simulink model "gm_spectrum_analyser"  (R2020a)
settings: Solver=VariableStepAuto  StartTime=0.0  StopTime=100000/256e6  RelTol=1e-3
InitFcn:
  | fs = 256e6;
undefined symbols (not defined in the file or in its folder): designMultirateFIR
libraries: hdlsllib x81, simulink x50, dspmlti4 x6, dsphdlxfrm x5, hdlmdlgenlib x4, dspswit3 x4, dspsigops x2, dspsigattribs x2
(part 1 of 5)
settings Model: Creator=david  LastModifiedBy=kevin
settings OptimizationCC: BlockReduction=off  ConditionallyExecuteInputs=off  DefaultParameterBehavior=Inlined
settings DebuggingCC: AlgebraicLoopMsg=error  InheritedTsInSrcMsg=none
settings HardwareCC: ProdBitPerPointer=32  ProdBitPerSizeT=32  ProdBitPerPtrDiffT=32  ProdLargestAtomicFloat=None  ProdIntDivRoundTo=Undefined  ProdEndianess=Unspecified  ProdWordSize=32  ProdHWDeviceType=ASIC/FPGA->ASIC/FPGA  TargetBitPerPointer=64  TargetBitPerSizeT=64  TargetBitPerPtrDiffT=64  TargetLongLongMode=on  TargetIntDivRoundTo=Zero  TargetEndianess=LittleEndian  TargetWordSize=64  TargetHWDeviceType=Custom Processor->MATLAB Host Computer  ProdEqTarget=off

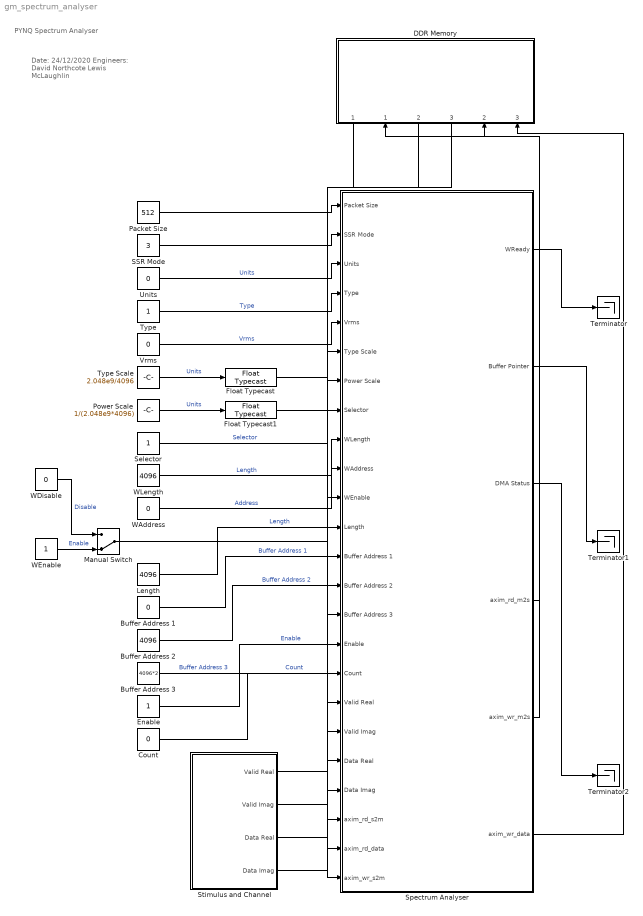
== system gm_spectrum_analyser ==
  note: PYNQ Spectrum Analyser
  note: Date:		24/12/2020
      | Engineers:	David Northcote
      | 			Lewis McLaughlin
  Buffer Address 1 : Constant  Value=0  OutDataTypeStr=uint32  SampleTime=1/fs
  Buffer Address 2 : Constant  Value=4096  OutDataTypeStr=uint32  SampleTime=1/fs
  Buffer Address 3 : Constant  Value=4096*2  OutDataTypeStr=uint32  SampleTime=1/fs
  Count : Constant  Value=0  OutDataTypeStr=uint32  SampleTime=1/fs
  DDR Memory : Subsystem
      settings: PortSchema="{\"entries\":[{\"content\":{\"sides\":[{\"content\":{\"connectorIds\":[]},\"type\":\"ConnectorPlacement.EquallySpacedRectSide\",\"uuid\":\"d9e4a1d3-1a90-455f-8481-c9ba23695512\"},{\"content\":{\"connectorIds\":[],\"side\":\"RIGHT\"},\"type\":\"ConnectorPlacement.EquallySpacedRectSide\",\"uuid\":\"d5cbf6c4-ca28-4b6e-a385-26c8d45a1027\"},{\"content\":{\"connectorIds\":[],\"side\":\"TOP\"},\"type\":\"ConnectorPlacement.EquallySpacedRectSide\",\"uuid\":\"1f61d25a-c781-4c7b-9600-adf853a1e7e2\"},{\"content\":{\"connectorIds\":[\"Out1\",\"In1\",\"Out2\",\"Out3\",\"In2\",\"In3\"],\"side\":\"BOTTOM\"},\"type\":\"ConnectorPlacement.EquallySpacedRectSide\",\"uuid\":\"b1131089-25c6-4639-a5ae-8f8dd9cc5fb0\"}]},\"type\":\"ConnectorPlacement.EquallySpacedConnector\",\"uuid\":\"baa6cdf8-4ad4-4b76-ad8b-23012dfe0a1e\"}],\"packageUris\":[\"http://schema.mathworks.com/mf0/Connector/19700101\"],\"version\":\"1.0\"}"
  Enable : Constant  OutDataTypeStr=uint32  SampleTime=1/fs
  Float Typecast : FloatTypecast
  Float Typecast1 : FloatTypecast
  Length : Constant  Value=4096  OutDataTypeStr=uint32  SampleTime=1/fs
  Manual Switch : ManualSwitch  CurrentSetting=0
  Packet Size : Constant  Value=512  OutDataTypeStr=uint32  SampleTime=-1
  Power Scale : Constant  Value=1/(2.048e9*4096)  OutDataTypeStr=single  SampleTime=-1
  SSR Mode : Constant  Value=3  OutDataTypeStr=uint32  SampleTime=-1
  Selector : Constant  OutDataTypeStr=uint32  SampleTime=-1
  Spectrum Analyser : Subsystem  TreatAsAtomicUnit=on
  Stimulus and Channel : Subsystem
  Terminator : Terminator
  Terminator1 : Terminator
  Terminator2 : Terminator
  Type : Constant  OutDataTypeStr=uint32  SampleTime=-1
  Type Scale : Constant  Value=2.048e9/4096  OutDataTypeStr=single  SampleTime=-1
  Units : Constant  Value=0  OutDataTypeStr=uint32  SampleTime=-1
  Vrms : Constant  Value=0  OutDataTypeStr=uint32  SampleTime=-1
  WAddress : Constant  Value=0  OutDataTypeStr=uint32  SampleTime=1/fs
  WDisable : Constant  Value=0  OutDataTypeStr=uint32  SampleTime=1/fs
  WEnable : Constant  OutDataTypeStr=uint32  SampleTime=1/fs
  WLength : Constant  Value=4096  OutDataTypeStr=uint32  SampleTime=1/fs
  wires:
  Spectrum Analyser/3(DMA Status) -> Terminator2/1
  Spectrum Analyser/2(Buffer Pointer) -> Terminator1/1
  Spectrum Analyser/1(WReady) -> Terminator/1
  Count/1 -> Spectrum Analyser/17(Count)  "Count"
  Enable/1 -> Spectrum Analyser/16(Enable)  "Enable"
  Buffer Address 2/1 -> Spectrum Analyser/14(Buffer Address 2)  "Buffer Address 2"
  Buffer Address 3/1 -> Spectrum Analyser/15(Buffer Address 3)  "Buffer Address 3"
  Buffer Address 1/1 -> Spectrum Analyser/13(Buffer Address 1)  "Buffer Address 1"
  Length/1 -> Spectrum Analyser/12(Length)  "Length"
  DDR Memory/3(axim_wr_s2m) -> Spectrum Analyser/24(axim_wr_s2m)
  DDR Memory/2(axim_rd_data) -> Spectrum Analyser/23(axim_rd_data)
  DDR Memory/1(axim_rd_s2m) -> Spectrum Analyser/22(axim_rd_s2m)
  Spectrum Analyser/6(axim_wr_data) -> DDR Memory/3(axim_wr_data)
  Spectrum Analyser/5(axim_wr_m2s) -> DDR Memory/2(axim_wr_m2s)
  Spectrum Analyser/4(axim_rd_m2s) -> DDR Memory/1(axim_rd_m2s)
  WLength/1 -> Spectrum Analyser/9(WLength)  "Length"
  WAddress/1 -> Spectrum Analyser/10(WAddress)  "Address"
  Manual Switch/1 -> Spectrum Analyser/11(WEnable)
  WDisable/1 -> Manual Switch/1  "Disable"
  WEnable/1 -> Manual Switch/2  "Enable"
  Packet Size/1 -> Spectrum Analyser/1(Packet Size)
  SSR Mode/1 -> Spectrum Analyser/2(SSR Mode)
  Selector/1 -> Spectrum Analyser/8(Selector)  "Selector"
  Power Scale/1 -> Float Typecast1/1  "Units"
  Float Typecast1/1 -> Spectrum Analyser/7(Power Scale)
  Float Typecast/1 -> Spectrum Analyser/6(Type Scale)
  Type Scale/1 -> Float Typecast/1  "Units"
  Units/1 -> Spectrum Analyser/3(Units)  "Units"
  Type/1 -> Spectrum Analyser/4(Type)  "Type"
  Vrms/1 -> Spectrum Analyser/5(Vrms)  "Vrms"
  Stimulus and Channel/4(Data Imag) -> Spectrum Analyser/21(Data Imag)
  Stimulus and Channel/3(Data Real) -> Spectrum Analyser/20(Data Real)
  Stimulus and Channel/2(Valid Imag) -> Spectrum Analyser/19(Valid Imag)
  Stimulus and Channel/1(Valid Real) -> Spectrum Analyser/18(Valid Real)

== system gm_spectrum_analyser/DDR Memory ==
  axim_rd_m2s : Inport
  axim_wr_m2s : Inport  Port=2
  axim_wr_data : Inport  Port=3
  AXI Read Interface Response Model : Subsystem
      settings: PortSchema="{\"entries\":[{\"content\":{\"sides\":[{\"content\":{\"connectorIds\":[]},\"type\":\"ConnectorPlacement.EquallySpacedRectSide\",\"uuid\":\"2b557e1e-8026-43d3-80e6-d6d80e534d60\"},{\"content\":{\"connectorIds\":[\"Out1\",\"In1\",\"Out2\"],\"side\":\"RIGHT\"},\"type\":\"ConnectorPlacement.EquallySpacedRectSide\",\"uuid\":\"d37ff7b5-bcab-46eb-bf2f-7b890d421095\"},{\"content\":{\"connectorIds\":[],\"side\":\"TOP\"},\"type\":\"ConnectorPlacement.EquallySpacedRectSide\",\"uuid\":\"b7392330-958c-44c2-9b9d-e2e6efc00005\"}]},\"type\":\"ConnectorPlacement.EquallySpacedConnector\",\"uuid\":\"d6fedbd7-9a1a-42de-85f8-78943e8230da\"}],\"packageUris\":[\"http://schema.mathworks.com/mf0/Connector/19700101\"],\"version\":\"1.0\"}"
  AXI Write Interface Response Model : Subsystem
      settings: PortSchema="{\"entries\":[{\"content\":{\"sides\":[{\"content\":{\"connectorIds\":[]},\"type\":\"ConnectorPlacement.EquallySpacedRectSide\",\"uuid\":\"6953abbe-a6d5-4686-b276-b89fe5e6bb23\"},{\"content\":{\"connectorIds\":[],\"side\":\"RIGHT\"},\"type\":\"ConnectorPlacement.EquallySpacedRectSide\",\"uuid\":\"539ff6ac-c243-4534-87d0-888ff9534a8b\"},{\"content\":{\"connectorIds\":[],\"side\":\"TOP\"},\"type\":\"ConnectorPlacement.EquallySpacedRectSide\",\"uuid\":\"8a126ba7-8eec-4733-ae4d-1ac2504ae558\"},{\"content\":{\"connectorIds\":[\"Out1\",\"In1\",\"In2\"],\"side\":\"BOTTOM\"},\"type\":\"ConnectorPlacement.EquallySpacedRectSide\",\"uuid\":\"05254abb-7168-4864-8cc1-53a55061df5a\"}]},\"type\":\"ConnectorPlacement.EquallySpacedConnector\",\"uuid\":\"821e8dd7-bdc5-437f-b697-1dcc78127ace\"}],\"packageUris\":[\"http://schema.mathworks.com/mf0/Connector/19700101\"],\"version\":\"1.0\"}"
  axim_rd_s2m : Outport
  axim_rd_data : Outport  Port=2
  axim_wr_s2m : Outport  Port=3
  wires:
  axim_wr_data/1 -> AXI Write Interface Response Model/2(axim_wr_data)
  AXI Read Interface Response Model/2(axim_rd_s2m) -> axim_rd_s2m/1  "axim_rd_s2m"
  axim_rd_m2s/1 -> AXI Read Interface Response Model/1(axim_rd_m2s)
  AXI Write Interface Response Model/1(axim_wr_s2m) -> axim_wr_s2m/1
  AXI Read Interface Response Model/1(axim_rd_data) -> axim_rd_data/1  "axim_rd_data"
  axim_wr_m2s/1 -> AXI Write Interface Response Model/1(axim_wr_m2s)

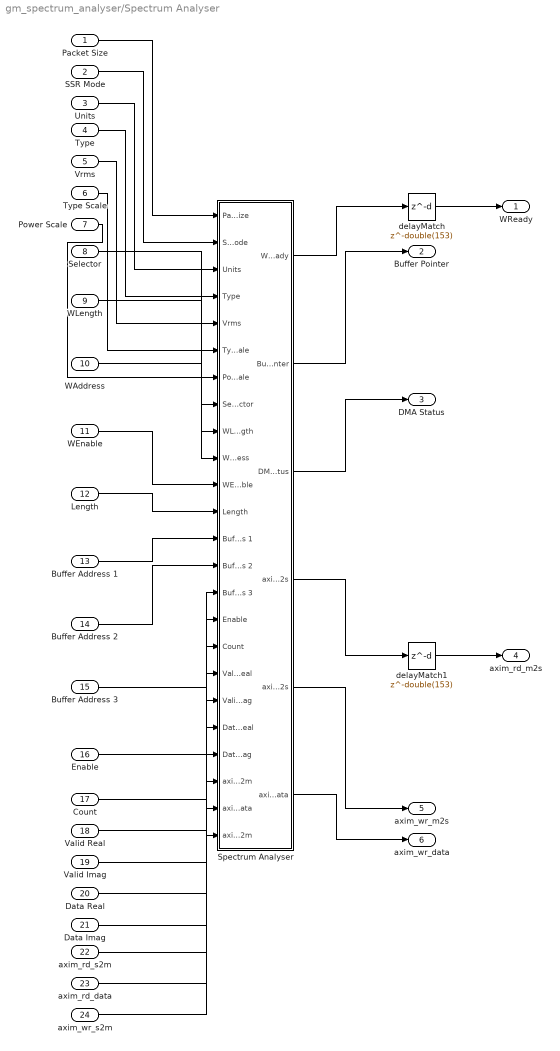
== system gm_spectrum_analyser/Spectrum Analyser ==
  Packet Size : Inport  OutDataTypeStr=uint32  PortDimensions=1  SampleTime=3.90625e-09
  SSR Mode : Inport  Port=2  OutDataTypeStr=uint32  PortDimensions=1  SampleTime=3.90625e-09
  Units : Inport  Port=3  OutDataTypeStr=uint32  PortDimensions=1  SampleTime=3.90625e-09
  Type : Inport  Port=4  OutDataTypeStr=uint32  PortDimensions=1  SampleTime=3.90625e-09
  Vrms : Inport  Port=5  OutDataTypeStr=uint32  PortDimensions=1  SampleTime=3.90625e-09
  Type Scale : Inport  Port=6  OutDataTypeStr=uint32  PortDimensions=1  SampleTime=3.90625e-09
  Power Scale : Inport  Port=7  OutDataTypeStr=uint32  PortDimensions=1  SampleTime=3.90625e-09
  Selector : Inport  Port=8  OutDataTypeStr=uint32  PortDimensions=1  SampleTime=3.90625e-09
  WLength : Inport  Port=9  OutDataTypeStr=uint32  PortDimensions=1  SampleTime=3.90625e-09
  WAddress : Inport  Port=10  OutDataTypeStr=uint32  PortDimensions=1  SampleTime=3.90625e-09
  WEnable : Inport  Port=11  OutDataTypeStr=uint32  PortDimensions=1  SampleTime=3.90625e-09
  Length : Inport  Port=12  OutDataTypeStr=uint32  PortDimensions=1  SampleTime=3.90625e-09
  Buffer Address 1 : Inport  Port=13  OutDataTypeStr=uint32  PortDimensions=1  SampleTime=3.90625e-09
  Buffer Address 2 : Inport  Port=14  OutDataTypeStr=uint32  PortDimensions=1  SampleTime=3.90625e-09
  Buffer Address 3 : Inport  Port=15  OutDataTypeStr=uint32  PortDimensions=1  SampleTime=3.90625e-09
  Enable : Inport  Port=16  OutDataTypeStr=uint32  PortDimensions=1  SampleTime=3.90625e-09
  Count : Inport  Port=17  OutDataTypeStr=uint32  PortDimensions=1  SampleTime=3.90625e-09
  Valid Real : Inport  Port=18  OutDataTypeStr=boolean  PortDimensions=1  SampleTime=3.90625e-09
  Valid Imag : Inport  Port=19  OutDataTypeStr=boolean  PortDimensions=1  SampleTime=3.90625e-09
  Data Real : Inport  Port=20  OutDataTypeStr=fixdt(0, 128, 0)  PortDimensions=1  SampleTime=3.90625e-09
  Data Imag : Inport  Port=21  OutDataTypeStr=fixdt(0, 128, 0)  PortDimensions=1  SampleTime=3.90625e-09
  axim_rd_s2m : Inport  Port=22  SampleTime=3.90625e-09
  axim_rd_data : Inport  Port=23  OutDataTypeStr=uint16  PortDimensions=1  SampleTime=3.90625e-09
  axim_wr_s2m : Inport  Port=24  SampleTime=3.90625e-09
  Spectrum Analyser : Subsystem
  delayMatch : Delay  DelayLength=double(153)  InitialCondition=0  SampleTime=3.90625e-09
  delayMatch1 : Delay  DelayLength=double(153)  InitialCondition=0  SampleTime=3.90625e-09
  WReady : Outport
  Buffer Pointer : Outport  Port=2
  DMA Status : Outport  Port=3
  axim_rd_m2s : Outport  Port=4
  axim_wr_m2s : Outport  Port=5
  axim_wr_data : Outport  Port=6
  wires:
  Packet Size/1 -> Spectrum Analyser/1(Packet Size)
  SSR Mode/1 -> Spectrum Analyser/2(SSR Mode)
  Units/1 -> Spectrum Analyser/3(Units)
  Type/1 -> Spectrum Analyser/4(Type)
  Vrms/1 -> Spectrum Analyser/5(Vrms)
  Type Scale/1 -> Spectrum Analyser/6(Type Scale)
  Power Scale/1 -> Spectrum Analyser/7(Power Scale)
  Selector/1 -> Spectrum Analyser/8(Selector)
  WLength/1 -> Spectrum Analyser/9(WLength)
  WAddress/1 -> Spectrum Analyser/10(WAddress)
  WEnable/1 -> Spectrum Analyser/11(WEnable)
  Length/1 -> Spectrum Analyser/12(Length)
  Buffer Address 1/1 -> Spectrum Analyser/13(Buffer Address 1)
  Buffer Address 2/1 -> Spectrum Analyser/14(Buffer Address 2)
  Buffer Address 3/1 -> Spectrum Analyser/15(Buffer Address 3)
  Enable/1 -> Spectrum Analyser/16(Enable)
  Count/1 -> Spectrum Analyser/17(Count)
  Valid Real/1 -> Spectrum Analyser/18(Valid Real)
  Valid Imag/1 -> Spectrum Analyser/19(Valid Imag)
  Data Real/1 -> Spectrum Analyser/20(Data Real)
  Data Imag/1 -> Spectrum Analyser/21(Data Imag)
  axim_rd_s2m/1 -> Spectrum Analyser/22(axim_rd_s2m)
  axim_rd_data/1 -> Spectrum Analyser/23(axim_rd_data)
  axim_wr_s2m/1 -> Spectrum Analyser/24(axim_wr_s2m)
  delayMatch/1 -> WReady/1
  Spectrum Analyser/2(Buffer Pointer) -> Buffer Pointer/1
  Spectrum Analyser/3(DMA Status) -> DMA Status/1
  delayMatch1/1 -> axim_rd_m2s/1
  Spectrum Analyser/5(axim_wr_m2s) -> axim_wr_m2s/1
  Spectrum Analyser/6(axim_wr_data) -> axim_wr_data/1
  Spectrum Analyser/1(WReady) -> delayMatch/1
  Spectrum Analyser/4(axim_rd_m2s) -> delayMatch1/1

== system gm_spectrum_analyser/Stimulus and Channel ==
  Channel : Subsystem
  Enable : Constant  OutDataTypeStr=boolean  SampleTime=-1
  Transmitter : Subsystem  TreatAsAtomicUnit=on
  Value : Constant  Value=hex2dec('7FFF7FFF')  OutDataTypeStr=uint32  SampleTime=-1
  Valid Real : Outport
  Valid Imag : Outport  Port=2
  Data Real : Outport  Port=3
  Data Imag : Outport  Port=4
  wires:
  Channel/2(Data Real) -> Data Real/1
  Channel/1(Valid Real) -> Valid Real/1
  Channel/4(Data Imag) -> Data Imag/1
  Channel/3(Valid Imag) -> Valid Imag/1
  Value/1 -> Transmitter/2(Value)  "Value"
  Transmitter/2(Data) -> Channel/2(Data)
  Transmitter/1(Valid) -> Channel/1(Valid)
  Enable/1 -> Transmitter/1(Enable)  "Enable"

== system gm_spectrum_analyser/DDR Memory/AXI Read Interface Response Model ==
  axim_rd_m2s : Inport
  Bus Creator : BusCreator  Inputs=2
  Bus Selector : BusSelector  OutputSignals=rd_addr,rd_len,rd_avalid
  Constant3 : Constant  OutDataTypeStr=boolean  SampleTime=-1
  DDR : Subsystem  mask{DDR_DATA=uint16(ones(1,4096)*2^15)}
      mask init:
      | %load('ram_data');
  axim_rd_data : Outport  VectorParamsAs1DForOutWhenUnconnected=off
  axim_rd_s2m : Outport  Port=2  VectorParamsAs1DForOutWhenUnconnected=off
  wires:
  Bus Creator/1 -> axim_rd_s2m/1
  DDR/1(rd_data) -> axim_rd_data/1  "rd_data"
  DDR/3(rd_dvalid) -> Bus Creator/2  "rd_dvalid"
  Constant3/1 -> DDR/4(rd_ready)
  Bus Selector/1 -> DDR/1(rd_addr)  "<rd_addr>"
  axim_rd_m2s/1 -> Bus Selector/1
  Bus Selector/3 -> DDR/3(rd_avalid)  "<rd_avalid>"
  DDR/2(rd_aready) -> Bus Creator/1  "rd_aready"
  Bus Selector/2 -> DDR/2(rd_len)  "<rd_len>"

== system gm_spectrum_analyser/DDR Memory/AXI Write Interface Response Model ==
  axim_wr_m2s : Inport
  axim_wr_data : Inport  Port=2
  AND : Logic  IconShape=distinctive  AllPortsSameDT=off  OutDataTypeStr=boolean
  Bus Creator2 : BusCreator  Inputs=2
  Bus Selector : BusSelector  OutputSignals=wr_valid
  Compare To Constant : simulink/Logic and Bit Operations/Compare To Constant  relop===  const=256  OutDataTypeStr=boolean
  Compare To Constant3 : simulink/Logic and Bit Operations/Compare To Constant  relop=<=  const=254  OutDataTypeStr=boolean
  Constant6 : Constant  Value=0  OutDataTypeStr=boolean  SampleTime=-1
  Delay : Delay  DelayLength=1  InitialCondition=0  UseCircularBuffer=on
  HDL Counter : hdlsllib/Sources/HDL Counter  CountType=Count limited  CountInit=0  CountStep=1  CountMax=256  CountFromType=Initial value  CountFrom=0  CountResetPort=off  CountLoadPort=off  CountEnbPort=on  CountDirPort=off  CountDataType=Unsigned  CountWordLen=10  CountFracLen=0  CountSampTime=1
  Manual Switch1 : ManualSwitch
  NOT : Logic  Operator=NOT  IconShape=distinctive  AllPortsSameDT=off  OutDataTypeStr=boolean
  OR : Logic  Operator=OR  IconShape=distinctive  AllPortsSameDT=off  OutDataTypeStr=boolean
  Serial to FFT Frame : Subsystem  mask{N=4096}
      mask prompts: N "FFT Size:"
      mask DialogControl DescGroupVar Prompt: Serial to FFT Frame
      mask DialogControl DescTextVar Prompt: This block converts serial FFT data to a frame of FFT data. An FFT shift is applied to correct for out of order FFT data.
      mask DialogControl ParameterGroupVar Prompt: Main
  Terminator : Terminator
  axim_wr_s2m : Outport
  wires:
  axim_wr_data/1 -> Serial to FFT Frame/2(Data In)
  Serial to FFT Frame/1(Data Out) -> Terminator/1
  axim_wr_m2s/1 -> Bus Selector/1
  Manual Switch1/1 -> Delay/1, Bus Creator2/1  "wr_ready"
  Bus Creator2/1 -> axim_wr_s2m/1  "axim_wr_s2m"
  NOT/1 -> OR/2
  OR/1 -> HDL Counter/1
  Compare To Constant3/1 -> Manual Switch1/1, NOT/1
  HDL Counter/1 -> Compare To Constant/1, Compare To Constant3/1
  Constant6/1 -> Manual Switch1/2
  AND/1 -> Serial to FFT Frame/1(Enable)
  Bus Selector/1 -> OR/1, AND/1  "<wr_valid>"
  Compare To Constant/1 -> Bus Creator2/2  "wr_complete"
  Delay/1 -> AND/2

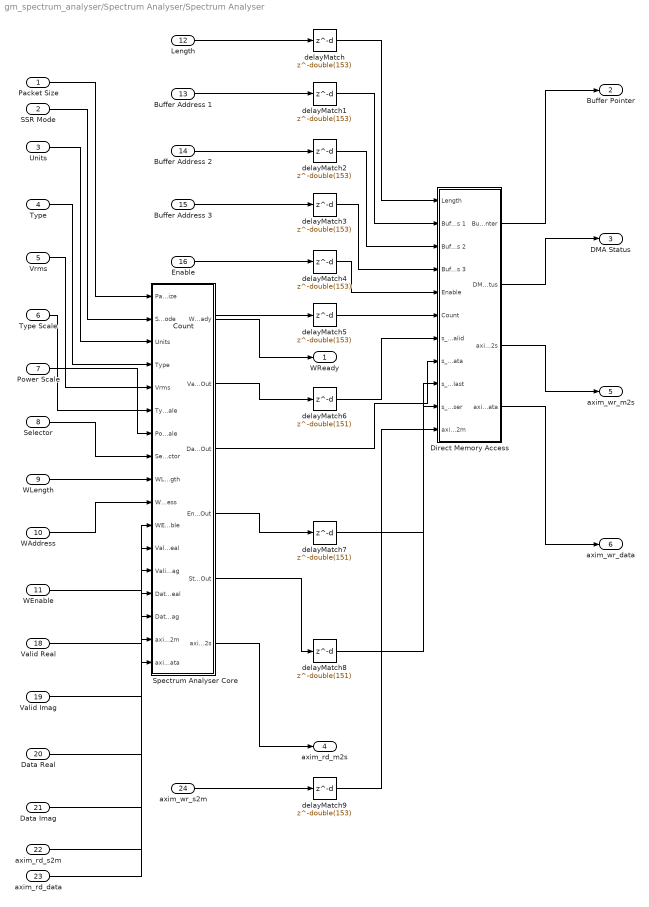
== system gm_spectrum_analyser/Spectrum Analyser/Spectrum Analyser ==
  Packet Size : Inport  OutDataTypeStr=uint32  SampleTime=3.90625e-09
  SSR Mode : Inport  Port=2  OutDataTypeStr=uint32  SampleTime=3.90625e-09
  Units : Inport  Port=3  OutDataTypeStr=uint32  SampleTime=3.90625e-09
  Type : Inport  Port=4  OutDataTypeStr=uint32  SampleTime=3.90625e-09
  Vrms : Inport  Port=5  OutDataTypeStr=uint32  SampleTime=3.90625e-09
  Type Scale : Inport  Port=6  OutDataTypeStr=uint32  SampleTime=3.90625e-09
  Power Scale : Inport  Port=7  OutDataTypeStr=uint32  SampleTime=3.90625e-09
  Selector : Inport  Port=8  OutDataTypeStr=uint32  SampleTime=3.90625e-09
  WLength : Inport  Port=9  OutDataTypeStr=uint32  SampleTime=3.90625e-09
  WAddress : Inport  Port=10  OutDataTypeStr=uint32  SampleTime=3.90625e-09
  WEnable : Inport  Port=11  OutDataTypeStr=uint32  SampleTime=3.90625e-09
  Length : Inport  Port=12  OutDataTypeStr=uint32  SampleTime=3.90625e-09
  Buffer Address 1 : Inport  Port=13  OutDataTypeStr=uint32  SampleTime=3.90625e-09
  Buffer Address 2 : Inport  Port=14  OutDataTypeStr=uint32  SampleTime=3.90625e-09
  Buffer Address 3 : Inport  Port=15  OutDataTypeStr=uint32  SampleTime=3.90625e-09
  Enable : Inport  Port=16  OutDataTypeStr=uint32  SampleTime=3.90625e-09
  Count : Inport  Port=17  OutDataTypeStr=uint32  SampleTime=3.90625e-09
  Valid Real : Inport  Port=18  OutDataTypeStr=boolean  SampleTime=3.90625e-09
  Valid Imag : Inport  Port=19  OutDataTypeStr=boolean  SampleTime=3.90625e-09
  Data Real : Inport  Port=20  OutDataTypeStr=fixdt(0, 128, 0)  SampleTime=3.90625e-09
  Data Imag : Inport  Port=21  OutDataTypeStr=fixdt(0, 128, 0)  SampleTime=3.90625e-09
  axim_rd_s2m : Inport  Port=22  SampleTime=3.90625e-09
  axim_rd_data : Inport  Port=23  OutDataTypeStr=uint16  SampleTime=3.90625e-09
  axim_wr_s2m : Inport  Port=24  SampleTime=3.90625e-09
  Direct Memory Access : Subsystem
  Spectrum Analyser Core : Subsystem
  delayMatch{,1..5,9} (7 alike) : Delay  DelayLength=double(153)  InitialCondition=0  SampleTime=3.90625e-09
  delayMatch6 : Delay  DelayLength=double(151)  InitialCondition=0  SampleTime=3.90625e-09
  delayMatch7 : Delay  DelayLength=double(151)  InitialCondition=0  SampleTime=3.90625e-09
  delayMatch8 : Delay  DelayLength=double(151)  InitialCondition=0  SampleTime=3.90625e-09
  WReady : Outport
  Buffer Pointer : Outport  Port=2
  DMA Status : Outport  Port=3
  axim_rd_m2s : Outport  Port=4
  axim_wr_m2s : Outport  Port=5
  axim_wr_data : Outport  Port=6
  wires:
  delayMatch/1 -> Direct Memory Access/1(Length)
  delayMatch1/1 -> Direct Memory Access/2(Buffer Address 1)
  delayMatch2/1 -> Direct Memory Access/3(Buffer Address 2)
  delayMatch3/1 -> Direct Memory Access/4(Buffer Address 3)
  delayMatch4/1 -> Direct Memory Access/5(Enable)
  delayMatch5/1 -> Direct Memory Access/6(Count)
  delayMatch9/1 -> Direct Memory Access/11(axim_wr_s2m)
  Direct Memory Access/1(Buffer Pointer) -> Buffer Pointer/1
  Direct Memory Access/2(DMA Status) -> DMA Status/1
  Direct Memory Access/3(axim_wr_m2s) -> axim_wr_m2s/1
  Direct Memory Access/4(axim_wr_data) -> axim_wr_data/1
  Spectrum Analyser Core/1(WReady) -> WReady/1
  delayMatch6/1 -> Direct Memory Access/7(s_axis_tvalid)
  Spectrum Analyser Core/3(Data Out) -> Direct Memory Access/8(s_axis_tdata)
  delayMatch7/1 -> Direct Memory Access/9(s_axis_tlast)
  delayMatch8/1 -> Direct Memory Access/10(s_axis_tuser)
  Spectrum Analyser Core/6(axim_rd_m2s) -> axim_rd_m2s/1
  Spectrum Analyser Core/2(Valid Out) -> delayMatch6/1
  Spectrum Analyser Core/4(End Out) -> delayMatch7/1
  Spectrum Analyser Core/5(Start Out) -> delayMatch8/1
  Packet Size/1 -> Spectrum Analyser Core/1(Packet Size)
  SSR Mode/1 -> Spectrum Analyser Core/2(SSR Mode)
  Units/1 -> Spectrum Analyser Core/3(Units)
  Type/1 -> Spectrum Analyser Core/4(Type)
  Vrms/1 -> Spectrum Analyser Core/5(Vrms)
  Type Scale/1 -> Spectrum Analyser Core/6(Type Scale)
  Power Scale/1 -> Spectrum Analyser Core/7(Power Scale)
  Selector/1 -> Spectrum Analyser Core/8(Selector)
  WLength/1 -> Spectrum Analyser Core/9(WLength)
  WAddress/1 -> Spectrum Analyser Core/10(WAddress)
  WEnable/1 -> Spectrum Analyser Core/11(WEnable)
  Length/1 -> delayMatch/1
  Buffer Address 1/1 -> delayMatch1/1
  Buffer Address 2/1 -> delayMatch2/1
  Buffer Address 3/1 -> delayMatch3/1
  Enable/1 -> delayMatch4/1
  Count/1 -> delayMatch5/1
  Valid Real/1 -> Spectrum Analyser Core/12(Valid Real)
  Valid Imag/1 -> Spectrum Analyser Core/13(Valid Imag)
  Data Real/1 -> Spectrum Analyser Core/14(Data Real)
  Data Imag/1 -> Spectrum Analyser Core/15(Data Imag)
  axim_rd_s2m/1 -> Spectrum Analyser Core/16(axim_rd_s2m)
  axim_rd_data/1 -> Spectrum Analyser Core/17(axim_rd_data)
  axim_wr_s2m/1 -> delayMatch9/1

== system gm_spectrum_analyser/Stimulus and Channel/Channel ==
  Valid : Inport
  Data : Inport  Port=2
  RF-ADC : Subsystem  mask{fs_ghz=4.096, decim=2x, ssr=8, mode=Fine, fc=0.256, fph=0, fcoarse=fs/4}
      mask prompts: fs_ghz "Sample Rate (GHz):"; decim "Interpolation Mode:"; ssr "Samples per AXI4-Stream Cycle:"; mode "Mixer Type:"; fc "NCO Frequency (GHz):"; fph "NCO Phase (Rads):"; fcoarse "Frequency:"
      mask init:
      | % Obtain the sample rate in Hz
      | fs = str2double(get_param(gcb, 'fs_ghz'))*1e9;
      | 
      | % Set the mode of the RF-DAC interpolation filter
      | switch get_param(gcb, 'decim')
      |     case '1x'
      |         D = 1;
      |     case '2x'
      |         D = 2;
      |     case '4x'
      |         D = 4;
      |     case '8x'
      |         D = 8;
      |     otherwise
      |         D = 1;
      | end
      | 
      | % Get the AXI-Stream clock for display to user
      | axi_clk = (fs/(str2double(get_param(gcb, 'ssr'))*D))*1e-6;
      | 
      | % Get the block mask object to manipulate settings
      | mo = get_param(gcb, 'MaskObject');
      | 
      | % Update text to display the required AXI-Stream clock
      | tc = mo.getDialogControl('axi_text');
      | tc.Prompt = ['      Required AXI-Stream Clock: ', num2str(axi_clk), ' MHz'];
      | 
      | % Set the RF-DAC Mixer mode
      | switch get_param(gcb, 'mode')
      |     case 'Bypass'
      |         m = 0;
      |     case 'Coarse'
      |         m = 1;
      |     case 'Fine'
      |         m = 2;
      |     otherwise
      |         m = 0;
      | end
      | 
      | % Set the RF-DAC Coarse Mixer mode
      | switch get_param(gcb, 'fcoarse')
      |     case 'fs/2'
      |         mc = 0;
      |     case 'fs/4'
      |         mc = 1;
      |     case '-fs/4'
      |         mc = 2;
      |     otherwise
      |         mc = 0;
      | end
      | 
      | % Set other blocks
      | set_param([gcb, '/Decimation Filter'], 'decim', get_param(gcb, 'decim'));
      mask Callback fs_ghz:
      | % Obtain the sample rate in Hz
      | fs = str2double(get_param(gcb, 'fs_ghz'))*1e9;
      | 
      | % Set the mode of the RF-DAC interpolation filter
      | switch get_param(gcb, 'decim')
      |     case '1x'
      |         D = 1;
      |     case '2x'
      |         D = 2;
      |     case '4x'
      |         D = 4;
      |     case '8x'
      |         D = 8;
      |     otherwise
      |         D = 1;
      | end
      | 
      | % Get the AXI-Stream clock for display to user
      | axi_clk = (fs/(str2double(get_param(gcb, 'ssr'))*D))*1e-6;
      | 
      | % Get the block mask object to manipulate settings
      | mo = get_param(gcb, 'MaskObject');
      | 
      | % Update text to display the required AXI-Stream clock
      | tc = mo.getDialogControl('axi_text');
      | tc.Prompt = ['      Required AXI-Stream Clock: ', num2str(axi_clk), ' MHz'];
      mask TypeOptions decim: 1x | 2x | 4x | 8x
      mask Callback decim:
      | % Obtain the sample rate in Hz
      | fs = str2double(get_param(gcb, 'fs_ghz'))*1e9;
      | 
      | % Set the mode of the RF-DAC interpolation filter
      | switch get_param(gcb, 'decim')
      |     case '1x'
      |         D = 1;
      |     case '2x'
      |         D = 2;
      |     case '4x'
      |         D = 4;
      |     case '8x'
      |         D = 8;
      |     otherwise
      |         D = 1;
      | end
      | 
      | % Get the AXI-Stream clock for display to user
      | axi_clk = (fs/(str2double(get_param(gcb, 'ssr'))*D))*1e-6;
      | 
      | % Get the block mask object to manipulate settings
      | mo = get_param(gcb, 'MaskObject');
      | 
      | % Update text to display the required AXI-Stream clock
      | tc = mo.getDialogControl('axi_text');
      | tc.Prompt = ['      Required AXI-Stream Clock: ', num2str(axi_clk), ' MHz'];
      mask TypeOptions ssr: 1 | 2 | 3 | 4 | 5 | 6 | 7 | 8 | 9 | 10 | 11 | 12 | 13 | 14 | 15 | 16
      mask Callback ssr:
      | % Obtain the sample rate in Hz
      | fs = str2double(get_param(gcb, 'fs_ghz'))*1e9;
      | 
      | % Set the mode of the RF-DAC interpolation filter
      | switch get_param(gcb, 'decim')
      |     case '1x'
      |         D = 1;
      |     case '2x'
      |         D = 2;
      |     case '4x'
      |         D = 4;
      |     case '8x'
      |         D = 8;
      |     otherwise
      |         D = 1;
      | end
      | 
      | % Get the AXI-Stream clock for display to user
      | axi_clk = (fs/(str2double(get_param(gcb, 'ssr'))*D))*1e-6;
      | 
      | % Get the block mask object to manipulate settings
      | mo = get_param(gcb, 'MaskObject');
      | 
      | % Update text to display the required AXI-Stream clock
      | tc = mo.getDialogControl('axi_text');
      | tc.Prompt = ['      Required AXI-Stream Clock: ', num2str(axi_clk), ' MHz'];
      mask TypeOptions mode: Coarse | Fine
      mask Callback mode:
      | % Get the block mask object to manipulate settings
      | mo = get_param(gcb, 'MaskObject');
      | 
      | % Hide group depending on Mixer mode choice
      | switch get_param(gcb, 'mode')
      |     case 'Bypass'
      |         mo.getDialogControl('coarse_group').Visible='off';
      |         mo.getDialogControl('mixer_group').Visible='off';
      |     case 'Coarse'
      |         mo.getDialogControl('coarse_group').Visible='on';
      |         mo.getDialogControl('mixer_group').Visible='off';
      |     case 'Fine'
      |         mo.getDialogControl('coarse_group').Visible='off';
      |         mo.getDialogControl('mixer_group').Visible='on';
      |     otherwise
      |         mo.getDialogControl('coarse_group').Visible='off';
      |         mo.getDialogControl('mixer_group').Visible='off';
      | end
      mask TypeOptions fcoarse: fs/2 | fs/4 | -fs/4
      mask DialogControl DescGroupVar Prompt: RF-DAC
      mask DialogControl DescTextVar Prompt: This block simulates one RF-ADC channel.
      mask DialogControl main_group Prompt: Data Settings
      mask DialogControl axi_text Prompt: Required AXI-Stream Clock: 256 MHz
      mask DialogControl Container5 Prompt: Mixer Settings
  RF-DAC : Subsystem  mask{fs_ghz=4.096, interp=4x, ssr=4, mode=Fine, fc=0.512, fph=0, fcoarse=fs/4}
      mask prompts: fs_ghz "Sample Rate (GHz):"; interp "Interpolation Mode:"; ssr "Samples per AXI4-Stream Cycle:"; mode "Mixer Type:"; fc "NCO Frequency (GHz):"; fph "NCO Phase (Rads):"; fcoarse "Frequency:"
      mask init:
      | % Obtain the sample rate in Hz
      | fs = str2double(get_param(gcb, 'fs_ghz'))*1e9;
      | 
      | % Set the mode of the RF-DAC interpolation filter
      | switch get_param(gcb, 'interp')
      |     case '1x'
      |         L = 1;
      |     case '2x'
      |         L = 2;
      |     case '4x'
      |         L = 4;
      |     case '8x'
      |         L = 8;
      |     otherwise
      |         L = 1;
      | end
      | 
      | % Get the AXI-Stream clock for display to user
      | axi_clk = (fs/(str2double(get_param(gcb, 'ssr'))*L))*1e-6;
      | 
      | % Get the block mask object to manipulate settings
      | mo = get_param(gcb, 'MaskObject');
      | 
      | % Update text to display the required AXI-Stream clock
      | tc = mo.getDialogControl('axi_text');
      | tc.Prompt = ['      Required AXI-Stream Clock: ', num2str(axi_clk), ' MHz'];
      | 
      | % Set the RF-DAC Mixer mode
      | switch get_param(gcb, 'mode')
      |     case 'Bypass'
      |         m = 0;
      |     case 'Coarse'
      |         m = 1;
      |     case 'Fine'
      |         m = 2;
      |     otherwise
      |         m = 0;
      | end
      | 
      | % Set the RF-DAC Coarse Mixer mode
      | switch get_param(gcb, 'fcoarse')
      |     case 'fs/2'
      |         mc = 0;
      |     case 'fs/4'
      |         mc = 1;
      |     case '-fs/4'
      |         mc = 2;
      |     otherwise
      |         mc = 0;
      | end
      | 
      | % Set other blocks
      | set_param([gcb, '/Interpolation Filter'], 'interp', get_param(gcb, 'interp'));
      mask Callback fs_ghz:
      | % Obtain the sample rate in Hz
      | fs = str2double(get_param(gcb, 'fs_ghz'))*1e9;
      | 
      | % Set the mode of the RF-DAC interpolation filter
      | switch get_param(gcb, 'interp')
      |     case '1x'
      |         L = 1;
      |     case '2x'
      |         L = 2;
      |     case '4x'
      |         L = 4;
      |     case '8x'
      |         L = 8;
      |     otherwise
      |         L = 1;
      | end
      | 
      | % Get the AXI-Stream clock for display to user
      | axi_clk = (fs/(str2double(get_param(gcb, 'ssr'))*L))*1e-6;
      | 
      | % Get the block mask object to manipulate settings
      | mo = get_param(gcb, 'MaskObject');
      | 
      | % Update text to display the required AXI-Stream clock
      | tc = mo.getDialogControl('axi_text');
      | tc.Prompt = ['      Required AXI-Stream Clock: ', num2str(axi_clk), ' MHz'];
      mask TypeOptions interp: 1x | 2x | 4x | 8x
      mask Callback interp:
      | % Obtain the sample rate in Hz
      | fs = str2double(get_param(gcb, 'fs_ghz'))*1e9;
      | 
      | % Set the mode of the RF-DAC interpolation filter
      | switch get_param(gcb, 'interp')
      |     case '1x'
      |         L = 1;
      |     case '2x'
      |         L = 2;
      |     case '4x'
      |         L = 4;
      |     case '8x'
      |         L = 8;
      |     otherwise
      |         L = 1;
      | end
      | 
      | % Get the AXI-Stream clock for display to user
      | axi_clk = (fs/(str2double(get_param(gcb, 'ssr'))*L))*1e-6;
      | 
      | % Get the block mask object to manipulate settings
      | mo = get_param(gcb, 'MaskObject');
      | 
      | % Update text to display the required AXI-Stream clock
      | tc = mo.getDialogControl('axi_text');
      | tc.Prompt = ['      Required AXI-Stream Clock: ', num2str(axi_clk), ' MHz'];
      mask TypeOptions ssr: 1 | 2 | 3 | 4 | 5 | 6 | 7 | 8 | 9 | 10 | 11 | 12 | 13 | 14 | 15 | 16
      mask Callback ssr:
      | % Obtain the sample rate in Hz
      | fs = str2double(get_param(gcb, 'fs_ghz'))*1e9;
      | 
      | % Set the mode of the RF-DAC interpolation filter
      | switch get_param(gcb, 'interp')
      |     case '1x'
      |         L = 1;
      |     case '2x'
      |         L = 2;
      |     case '4x'
      |         L = 4;
      |     case '8x'
      |         L = 8;
      |     otherwise
      |         L = 1;
      | end
      | 
      | % Get the AXI-Stream clock for display to user
      | axi_clk = (fs/(str2double(get_param(gcb, 'ssr'))*L))*1e-6;
      | 
      | % Get the block mask object to manipulate settings
      | mo = get_param(gcb, 'MaskObject');
      | 
      | % Update text to display the required AXI-Stream clock
      | tc = mo.getDialogControl('axi_text');
      | tc.Prompt = ['      Required AXI-Stream Clock: ', num2str(axi_clk), ' MHz'];
      mask TypeOptions mode: Coarse | Fine
      mask Callback mode:
      | % Get the block mask object to manipulate settings
      | mo = get_param(gcb, 'MaskObject');
      | 
      | % Hide group depending on Mixer mode choice
      | switch get_param(gcb, 'mode')
      |     case 'Bypass'
      |         mo.getDialogControl('coarse_group').Visible='off';
      |         mo.getDialogControl('mixer_group').Visible='off';
      |     case 'Coarse'
      |         mo.getDialogControl('coarse_group').Visible='on';
      |         mo.getDialogControl('mixer_group').Visible='off';
      |     case 'Fine'
      |         mo.getDialogControl('coarse_group').Visible='off';
      |         mo.getDialogControl('mixer_group').Visible='on';
      |     otherwise
      |         mo.getDialogControl('coarse_group').Visible='off';
      |         mo.getDialogControl('mixer_group').Visible='off';
      | end
      mask TypeOptions fcoarse: fs/2 | fs/4 | -fs/4
      mask DialogControl DescGroupVar Prompt: RF-DAC
      mask DialogControl DescTextVar Prompt: This block simulates one RF-DAC channel.
      mask DialogControl main_group Prompt: Data Settings
      mask DialogControl axi_text Prompt: Required AXI-Stream Clock: 256 MHz
      mask DialogControl Container5 Prompt: Mixer Settings
  RX RF Balun : Gain  Gain=1/2
  TX RF Balun : Gain  Gain=1/2
  Valid Real : Outport
  Data Real : Outport  Port=2
  Valid Imag : Outport  Port=3
  Data Imag : Outport  Port=4
  wires:
  RF-ADC/2(Valid Imag) -> Valid Imag/1
  RF-DAC/1(Data Out) -> TX RF Balun/1
  RF-ADC/1(Valid Real) -> Valid Real/1
  RF-ADC/4(Data Imag) -> Data Imag/1
  Data/1 -> RF-DAC/2(Data)
  RX RF Balun/1 -> RF-ADC/1(Data In)
  RF-ADC/3(Data Real) -> Data Real/1
  Valid/1 -> RF-DAC/1(Valid)
  TX RF Balun/1 -> RX RF Balun/1

== system gm_spectrum_analyser/Stimulus and Channel/Transmitter ==
  Enable : Inport
  Value : Inport  Port=2
  Transmitter : Subsystem  TreatAsAtomicUnit=on
  Valid : Outport
  Data : Outport  Port=2
  wires:
  Value/1 -> Transmitter/2(Value)
  Enable/1 -> Transmitter/1(Enable)
  Transmitter/1(Valid) -> Valid/1
  Transmitter/2(Data) -> Data/1

== system gm_spectrum_analyser/DDR Memory/AXI Read Interface Response Model/DDR ==
  rd_addr : Inport
  rd_len : Inport  Port=2
  rd_avalid : Inport  Port=3
  rd_ready : Inport  Port=4
  Delay : Delay  DelayLength=3
  Delay1 : Delay  DelayLength=3
  Delay2 : Delay  DelayLength=1
  Enabled Subsystem : Subsystem  TreatAsAtomicUnit=on
  rd_data : Outport  VectorParamsAs1DForOutWhenUnconnected=off
  rd_aready : Outport  Port=2  VectorParamsAs1DForOutWhenUnconnected=off
  rd_dvalid : Outport  Port=3  VectorParamsAs1DForOutWhenUnconnected=off
  wires:
  Delay2/1 -> rd_aready/1
  Delay1/1 -> rd_dvalid/1
  Enabled Subsystem/3(rd_dvalid) -> Delay1/1  "rd_dvalid"
  rd_ready/1 -> Enabled Subsystem/Enable
  Enabled Subsystem/2(rd_aready) -> Delay2/1  "rd_ack"
  rd_avalid/1 -> Enabled Subsystem/3(rd_avalid)
  Delay/1 -> rd_data/1
  Enabled Subsystem/1(rd_data) -> Delay/1  "rd_data"
  rd_len/1 -> Enabled Subsystem/2(rd_len)
  rd_addr/1 -> Enabled Subsystem/1(rd_addr)

== system gm_spectrum_analyser/DDR Memory/AXI Write Interface Response Model/Serial to FFT Frame ==
  Enable : Inport
  Data In : Inport  Port=2
  Enabled Subsystem2 : Subsystem  TreatAsAtomicUnit=on
  Float Typecast : FloatTypecast
  Data Out : Outport
  wires:
  Enabled Subsystem2/1(Data Out) -> Float Typecast/1
  Enable/1 -> Enabled Subsystem2/Enable
  Data In/1 -> Enabled Subsystem2/1(Data In)
  Float Typecast/1 -> Data Out/1

== system gm_spectrum_analyser/Spectrum Analyser/Spectrum Analyser/Direct Memory Access ==
  Length : Inport  OutDataTypeStr=uint32  SampleTime=3.90625e-09
  Buffer Address 1 : Inport  Port=2  OutDataTypeStr=uint32  SampleTime=3.90625e-09
  Buffer Address 2 : Inport  Port=3  OutDataTypeStr=uint32  SampleTime=3.90625e-09
  Buffer Address 3 : Inport  Port=4  OutDataTypeStr=uint32  SampleTime=3.90625e-09
  Enable : Inport  Port=5  OutDataTypeStr=uint32  SampleTime=3.90625e-09
  Count : Inport  Port=6  OutDataTypeStr=uint32  SampleTime=3.90625e-09
  s_axis_tvalid : Inport  Port=7  OutDataTypeStr=boolean  SampleTime=3.90625e-09
  s_axis_tdata : Inport  Port=8  OutDataTypeStr=uint32  SampleTime=3.90625e-09
  s_axis_tlast : Inport  Port=9  OutDataTypeStr=boolean  SampleTime=3.90625e-09
  s_axis_tuser : Inport  Port=10  OutDataTypeStr=boolean  SampleTime=3.90625e-09
  axim_wr_s2m : Inport  Port=11  SampleTime=3.90625e-09
  Direct Memory Access : Subsystem
  Buffer Pointer : Outport
  DMA Status : Outport  Port=2
  axim_wr_m2s : Outport  Port=3
  axim_wr_data : Outport  Port=4
  wires:
  Direct Memory Access/1(wr_data) -> axim_wr_data/1
  Direct Memory Access/2(wr_m2s) -> axim_wr_m2s/1
  Direct Memory Access/3(Buffer Pointer) -> Buffer Pointer/1
  Direct Memory Access/4(DMA Status) -> DMA Status/1
  Length/1 -> Direct Memory Access/1(Length)
  Buffer Address 1/1 -> Direct Memory Access/3(Buffer Address 1)
  Buffer Address 2/1 -> Direct Memory Access/4(Buffer Address 2)
  Buffer Address 3/1 -> Direct Memory Access/5(Buffer Address 3)
  Enable/1 -> Direct Memory Access/6(Enable DMA)
  Count/1 -> Direct Memory Access/2(Count)
  s_axis_tvalid/1 -> Direct Memory Access/7(Valid In)
  s_axis_tdata/1 -> Direct Memory Access/8(Data In)
  s_axis_tlast/1 -> Direct Memory Access/10(End In)
  s_axis_tuser/1 -> Direct Memory Access/9(Start In)
  axim_wr_s2m/1 -> Direct Memory Access/11(wr_ready)

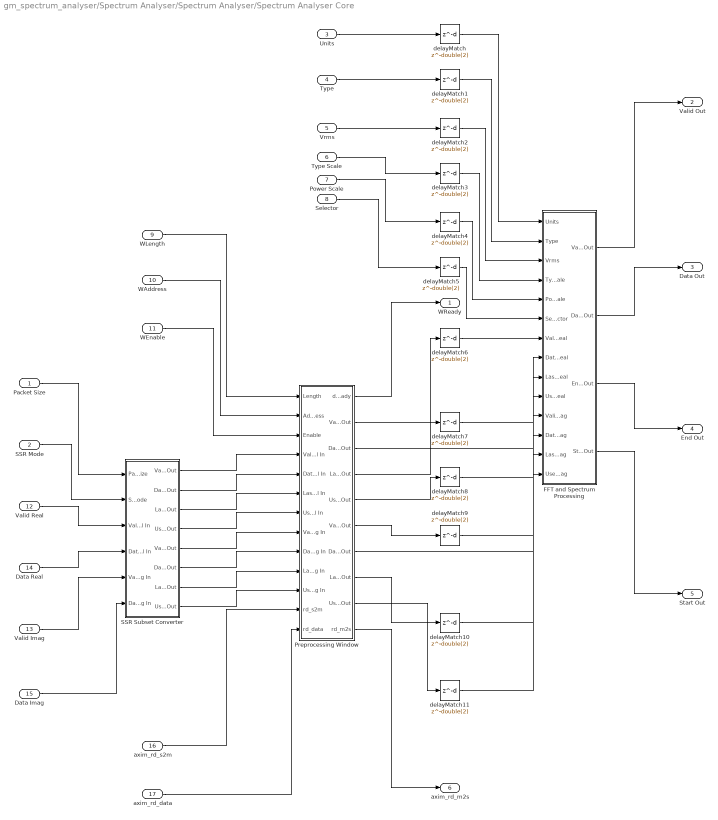
== system gm_spectrum_analyser/Spectrum Analyser/Spectrum Analyser/Spectrum Analyser Core ==
  Packet Size : Inport  OutDataTypeStr=uint32  SampleTime=3.90625e-09
  SSR Mode : Inport  Port=2  OutDataTypeStr=uint32  SampleTime=3.90625e-09
  Units : Inport  Port=3  OutDataTypeStr=uint32  SampleTime=3.90625e-09
  Type : Inport  Port=4  OutDataTypeStr=uint32  SampleTime=3.90625e-09
  Vrms : Inport  Port=5  OutDataTypeStr=uint32  SampleTime=3.90625e-09
  Type Scale : Inport  Port=6  OutDataTypeStr=uint32  SampleTime=3.90625e-09
  Power Scale : Inport  Port=7  OutDataTypeStr=uint32  SampleTime=3.90625e-09
  Selector : Inport  Port=8  OutDataTypeStr=uint32  SampleTime=3.90625e-09
  WLength : Inport  Port=9  OutDataTypeStr=uint32  SampleTime=3.90625e-09
  WAddress : Inport  Port=10  OutDataTypeStr=uint32  SampleTime=3.90625e-09
  WEnable : Inport  Port=11  OutDataTypeStr=uint32  SampleTime=3.90625e-09
  Valid Real : Inport  Port=12  OutDataTypeStr=boolean  SampleTime=3.90625e-09
  Valid Imag : Inport  Port=13  OutDataTypeStr=boolean  SampleTime=3.90625e-09
  Data Real : Inport  Port=14  OutDataTypeStr=fixdt(0, 128, 0)  SampleTime=3.90625e-09
  Data Imag : Inport  Port=15  OutDataTypeStr=fixdt(0, 128, 0)  SampleTime=3.90625e-09
  axim_rd_s2m : Inport  Port=16  SampleTime=3.90625e-09
  axim_rd_data : Inport  Port=17  OutDataTypeStr=uint16  SampleTime=3.90625e-09
  FFT and Spectrum Processing : Subsystem
  Preprocessing Window : Subsystem
  SSR Subset Converter : Subsystem
  delayMatch{,1..11} (12 alike) : Delay  DelayLength=double(2)  InitialCondition=0  SampleTime=3.90625e-09
  WReady : Outport
  Valid Out : Outport  Port=2
  Data Out : Outport  Port=3
  End Out : Outport  Port=4
  Start Out : Outport  Port=5
  axim_rd_m2s : Outport  Port=6
  wires:
  delayMatch/1 -> FFT and Spectrum Processing/1(Units)
  delayMatch1/1 -> FFT and Spectrum Processing/2(Type)
  delayMatch2/1 -> FFT and Spectrum Processing/3(Vrms)
  delayMatch3/1 -> FFT and Spectrum Processing/4(Type Scale)
  delayMatch4/1 -> FFT and Spectrum Processing/5(Power Scale)
  delayMatch5/1 -> FFT and Spectrum Processing/6(Selector)
  FFT and Spectrum Processing/1(Valid Out) -> Valid Out/1
  FFT and Spectrum Processing/2(Data Out) -> Data Out/1
  FFT and Spectrum Processing/3(End Out) -> End Out/1
  FFT and Spectrum Processing/4(Start Out) -> Start Out/1
  Preprocessing Window/1(dma_ready) -> WReady/1
  delayMatch6/1 -> FFT and Spectrum Processing/7(Valid Real)
  Preprocessing Window/3(Data Real Out) -> FFT and Spectrum Processing/8(Data Real)
  delayMatch7/1 -> FFT and Spectrum Processing/9(Last Real)
  delayMatch8/1 -> FFT and Spectrum Processing/10(User Real)
  delayMatch9/1 -> FFT and Spectrum Processing/11(Valid Imag)
  Preprocessing Window/7(Data Imag Out) -> FFT and Spectrum Processing/12(Data Imag)
  delayMatch10/1 -> FFT and Spectrum Processing/13(Last Imag)
  delayMatch11/1 -> FFT and Spectrum Processing/14(User Imag)
  Preprocessing Window/10(rd_m2s) -> axim_rd_m2s/1
  SSR Subset Converter/1(Valid Real Out) -> Preprocessing Window/4(Valid Real In)
  SSR Subset Converter/2(Data Real Out) -> Preprocessing Window/5(Data Real In)
  SSR Subset Converter/3(Last Real Out) -> Preprocessing Window/6(Last Real In)
  SSR Subset Converter/4(User Real Out) -> Preprocessing Window/7(User Real In)
  SSR Subset Converter/5(Valid Imag Out) -> Preprocessing Window/8(Valid Imag In)
  SSR Subset Converter/6(Data Imag Out) -> Preprocessing Window/9(Data Imag In)
  SSR Subset Converter/7(Last Imag Out) -> Preprocessing Window/10(Last Imag In)
  SSR Subset Converter/8(User Imag Out) -> Preprocessing Window/11(User Imag In)
  Preprocessing Window/2(Valid Real Out) -> delayMatch6/1
  Preprocessing Window/4(Last Real Out) -> delayMatch7/1
  Preprocessing Window/5(User Real Out) -> delayMatch8/1
  Preprocessing Window/6(Valid Imag Out) -> delayMatch9/1
  Preprocessing Window/8(Last Imag Out) -> delayMatch10/1
  Preprocessing Window/9(User Imag Out) -> delayMatch11/1
  Packet Size/1 -> SSR Subset Converter/1(Packet Size)
  SSR Mode/1 -> SSR Subset Converter/2(SSR Mode)
  Units/1 -> delayMatch/1
  Type/1 -> delayMatch1/1
  Vrms/1 -> delayMatch2/1
  Type Scale/1 -> delayMatch3/1
  Power Scale/1 -> delayMatch4/1
  Selector/1 -> delayMatch5/1
  WLength/1 -> Preprocessing Window/1(Length)
  WAddress/1 -> Preprocessing Window/2(Address)
  WEnable/1 -> Preprocessing Window/3(Enable)
  Valid Real/1 -> SSR Subset Converter/3(Valid Real In)
  Valid Imag/1 -> SSR Subset Converter/5(Valid Imag In)
  Data Real/1 -> SSR Subset Converter/4(Data Real In)
  Data Imag/1 -> SSR Subset Converter/6(Data Imag In)
  axim_rd_s2m/1 -> Preprocessing Window/12(rd_s2m)
  axim_rd_data/1 -> Preprocessing Window/13(rd_data)

== system gm_spectrum_analyser/Stimulus and Channel/Channel/RF-ADC ==
  Data In : Inport
  Complex to Real-Imag : ComplexToRealImag
  Decimation Filter : Subsystem  mask{decim=2x}
      mask prompts: decim "Decimation Factor:"
      mask init:
      | fir0 = dsp.FIRDecimator('DecimationFactor', 2,...
      |                            'CoefficientsDataType', 'Custom',...
      |                            'CustomCoefficientsDataType', numerictype([], 16, 14),...
      |                            'FullPrecisionOverride', false,...
      |                            'OutputDataType', 'Custom',...
      |                            'CustomOutputDataType', numerictype([], 16, 15),...
      |                            'Numerator', [-6, 0 54, 0, -254, 0, 1230, 2048, 1230, 0, -254, 0, 54, 0, -6]/2048);
      | fir1 = dsp.FIRDecimator('DecimationFactor', 2,...
      |                            'CoefficientsDataType', 'Custom',...
      |                            'CustomCoefficientsDataType', numerictype([], 16, 14),...
      |                            'FullPrecisionOverride', false,...
      |                            'OutputDataType', 'Custom',...
      |                            'CustomOutputDataType', numerictype([], 16, 15),...
      |                            'Numerator', [-12, 0, 84, 0, -337, 0, 1008, 0, -2693, 0, 10142, 16384, 10142, 0, -2693, 0, 1008, 0, -337, 0, 84, 0 ,-12]/16384);
      | fir2 = dsp.FIRDecimator('DecimationFactor', 2,...
      |                            'CoefficientsDataType', 'Custom',...
      |                            'CustomCoefficientsDataType', numerictype([], 16, 14),...
      |                            'FullPrecisionOverride', false,...
      |                            'OutputDataType', 'Custom',...
      |                            'CustomOutputDataType', numerictype([], 16, 15),...
      |                            'Numerator', [5, 0, -17, 0, 44, 0, -96, 0, 187, 0, -335, 0, 565, 0, -906, 0, 1401, 0, -2112, 0, 3145, 0, -4723, 0, 7415, 0, -13331, 0, 41526, 65536, 41526, 0, -13331, 0, 7415, 0, -4723, 0, 3145, 0, -2112, 0, 1401, 0, -906, 0, 565, 0, -335, 0, 187, 0, -96, 0, 44, 0, -17, 0, 5]/65536);
      | switch get_param(gcb, 'decim')
      |     case '1x'
      |         if ~strcmp(get_param([gcb, '/FIR 0'], 'Commented'), 'through')
      |             set_param([gcb, '/FIR 0'],'Commented','through');
      |         end
      |         
      |         if ~strcmp(get_param([gcb, '/FIR 1'], 'Commented'), 'through')
      |             set_param([gcb, '/FIR 1'],'Commented','through');
      |         end
      |         
      |         if ~strcmp(get_param([gcb, '/FIR 2'], 'Commented'), 'through')
      |             set_param([gcb, '/FIR 2'],'Commented','through');
      |         end
      |             
      |     case '2x'
      |         if ~strcmp(get_param([gcb, '/FIR 0'], 'Commented'), 'off')
      |             set_param([gcb, '/FIR 0'],'Commented','through');
      |         end
      |         
      |         if ~strcmp(get_param([gcb, '/FIR 1'], 'Commented'), 'through')
      |             set_param([gcb, '/FIR 1'],'Commented','through');
      |         end
      |         
      |         if ~strcmp(get_param([gcb, '/FIR 2'], 'Commented'), 'through')
      |             set_param([gcb, '/FIR 2'],'Commented','off');
      |         end
      | 
      |     case '4x'
      |         if ~strcmp(get_param([gcb, '/FIR 0'], 'Commented'), 'off')
      |             set_param([gcb, '/FIR 0'],'Commented','through');
      |         end
      |         
      |         if ~strcmp(get_param([gcb, '/FIR 1'], 'Commented'), 'off')
      |             set_param([gcb, '/FIR 1'],'Commented','off');
      |         end
      |         
      |         if ~strcmp(get_param([gcb, '/FIR 2'], 'Commented'), 'through')
      |             set_param([gcb, '/FIR 2'],'Commented','off');
      |         end
      |         
      |     case '8x'
      |         if ~strcmp(get_param([gcb, '/FIR 0'], 'Commented'), 'off')
      |             set_param([gcb, '/FIR 0'],'Commented','off');
      |         end
      |         
      |         if ~strcmp(get_param([gcb, '/FIR 1'], 'Commented'), 'off')
      |             set_param([gcb, '/FIR 1'],'Commented','off');
      |         end
      |         
      |         if ~strcmp(get_param([gcb, '/FIR 2'], 'Commented'), 'off')
      |             set_param([gcb, '/FIR 2'],'Commented','off');
      |         end
      | 
      | end
      mask TypeOptions decim: 1x | 2x | 4x | 8x
      mask DialogControl DescGroupVar Prompt: RF-DAC Interpolation Filter
      mask DialogControl DescTextVar Prompt: This block simulates the RF-DAC interpolation stage using the same coefficients stored in the interpolation filters.
      mask DialogControl ParameterGroupVar Prompt: Main
  NCO and Mixer : Subsystem
  RF-ADC : Subsystem
  SSR Converter RF-ADC : Subsystem
  Valid Real : Outport  VectorParamsAs1DForOutWhenUnconnected=off
  Valid Imag : Outport  Port=2  VectorParamsAs1DForOutWhenUnconnected=off
  Data Real : Outport  Port=3  VectorParamsAs1DForOutWhenUnconnected=off
  Data Imag : Outport  Port=4  VectorParamsAs1DForOutWhenUnconnected=off
  wires:
  NCO and Mixer/1(Data Out) -> Decimation Filter/1(Data In)
  RF-ADC/1(Data Out) -> NCO and Mixer/1(Data In)
  Data In/1 -> RF-ADC/1(Data In)
  Decimation Filter/1(Data Out) -> Complex to Real-Imag/1
  Complex to Real-Imag/1 -> SSR Converter RF-ADC/1(Real In)
  Complex to Real-Imag/2 -> SSR Converter RF-ADC/2(Imag In)
  SSR Converter RF-ADC/4(Imag Out) -> Data Imag/1
  SSR Converter RF-ADC/3(Real Out) -> Data Real/1
  SSR Converter RF-ADC/1(Valid Real) -> Valid Real/1
  SSR Converter RF-ADC/2(Valid Imag) -> Valid Imag/1
